simulink model "evap_simscape"  (R2023b)
settings: Solver=VariableStepAuto  StartTime=0.0  StopTime=eTime  RelTol=1e-3
values from neighbouring files (symbols this model uses):
  initial = struct()    [evap_simscape_code.m]
undefined symbols (not defined in the file or in its folder): refProp
libraries: nesl_utility x39, fl_lib x24, SimscapeFluids_lib x3
settings Model: Creator=jisung  LastModifiedBy=jisung
settings OptimizationCC: OptimizeBlockIOStorage=off  OptimizeDataStoreBuffers=off  BusAssignmentInplaceUpdate=off
settings DebuggingCC: SFUnexpectedBacktrackingDiag=warning  SFNoUnconditionalDefaultTransitionDiag=warning
settings RTWCC: GenCodeOnly=on  GenerateReport=on  Toolchain=Microsoft Visual C++ 2022 v17.0 | nmake (64-bit Windows)  BuildConfiguration=Debug  LaunchReport=on  TargetLang=C++
settings CodeAppCC: ForceParamTrailComments=on  MATLABSourceComments=on  EnableCustomComments=on
settings GRTTargetCC: TargetLangStandard=C++11 (ISO)  CombineSignalStateStructs=on  CodeInterfacePackaging=Reusable function  SupportVariableSizeSignals=on  GenerateAllocFcn=on  MultiInstanceErrorCode=Warning

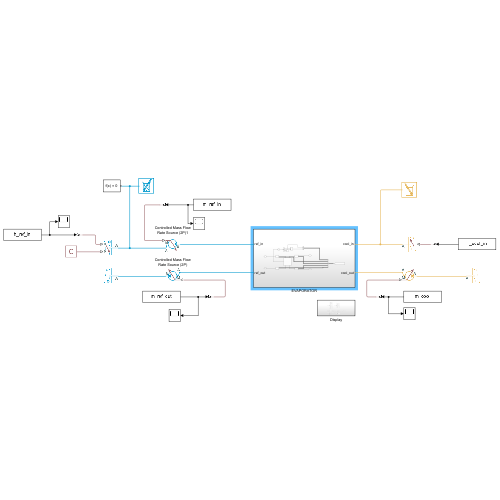
[thumbnail: Simulink's stored preview of the top-level diagram]
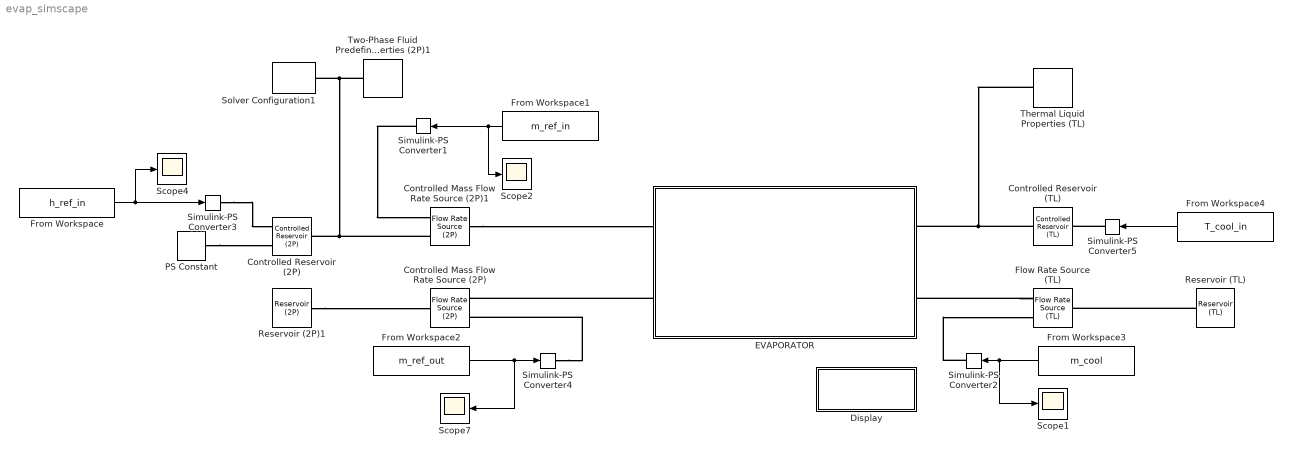
== system evap_simscape ==
  Controlled Mass Flow Rate Source (2P) : fl_lib/Two-Phase Fluid/Sources/Flow Rate Source (2P)  source_type=foundation.enum.constant_controlled.controlled  flow_type=foundation.enum.mass_volumetric_flow.mass  mass_flow=0 kg/s  volumetric_flow=0 m^3/s  power_spec=foundation.enum.power_spec.isentropic  area_A=pi * 12^2 / 4 mm^2  area_B=pi * 12^2 / 4 mm^2
      settings: InternalSimscapePortConfiguration="{\"Bottom\":[],\"Left\":[{\"id\":\"A\",\"label\":\"A\",\"type\":\"foundation.two_phase_fluid.two_phase_fluid\"},{\"id\":\"M\",\"label\":\"M\",\"type\":\"input\"}],\"Right\":[{\"id\":\"B\",\"label\":\"B\",\"type\":\"foundation.two_phase_fluid.two_phase_fluid\"}],\"Top\":[]}"
  Controlled Mass Flow Rate Source (2P)1 : fl_lib/Two-Phase Fluid/Sources/Flow Rate Source (2P)  source_type=foundation.enum.constant_controlled.controlled  flow_type=foundation.enum.mass_volumetric_flow.mass  mass_flow=0 kg/s  volumetric_flow=0 m^3/s  power_spec=foundation.enum.power_spec.isentropic  area_A=pi * 12^2 / 4 mm^2  area_B=pi * 12^2 / 4 mm^2
      settings: InternalSimscapePortConfiguration="{\"Bottom\":[],\"Left\":[{\"id\":\"A\",\"label\":\"A\",\"type\":\"foundation.two_phase_fluid.two_phase_fluid\"},{\"id\":\"M\",\"label\":\"M\",\"type\":\"input\"}],\"Right\":[{\"id\":\"B\",\"label\":\"B\",\"type\":\"foundation.two_phase_fluid.two_phase_fluid\"}],\"Top\":[]}"
  Controlled Reservoir (2P) : fl_lib/Two-Phase Fluid/Elements/Controlled Reservoir (2P)  pressure_spec=foundation.enum.ControlledReservoirPressureSpec2P.Specified  energy_spec=foundation.enum.ControlledReservoirEnergySpec2P.Enthalpy  area_A=0.01 m^2  pressure_limit_spec=foundation.enum.PressureLimitSpec2P.Warn
      settings: InternalSimscapePortConfiguration="{\"Bottom\":[],\"Left\":[{\"id\":\"A\",\"label\":\"A\",\"type\":\"foundation.two_phase_fluid.two_phase_fluid\"}],\"Right\":[{\"id\":\"H\",\"label\":\"H\",\"type\":\"input\"},{\"id\":\"P\",\"label\":\"P\",\"type\":\"input\"}],\"Top\":[]}"
  Controlled Reservoir (TL) : fl_lib/Thermal Liquid/Elements/Controlled Reservoir (TL)  pressure_spec=foundation.enum.pressure_spec.atmospheric  reservoir_pressure=0.101325 MPa  area=0.01 m^2
      settings: InternalSimscapePortConfiguration="{\"Bottom\":[],\"Left\":[{\"id\":\"A\",\"label\":\"A\",\"type\":\"foundation.thermal_liquid.thermal_liquid\"}],\"Right\":[{\"id\":\"T_in\",\"label\":\"T\",\"type\":\"input\"}],\"Top\":[]}"
  Display : Subsystem
  EVAPORATOR : Subsystem
  Flow Rate Source (TL) : fl_lib/Thermal Liquid/Sources/Flow Rate Source (TL)  source_type=foundation.enum.constant_controlled.controlled  flow_type=foundation.enum.mass_volumetric_flow.mass  mass_flow=0 kg/s  volumetric_flow=0 m^3/s  power_spec=foundation.enum.power_spec.isentropic  area=0.01 m^2
  From Workspace : FromWorkspace  VariableName=h_ref_in  Interpolate=off  OutputAfterFinalValue=Holding final value
  From Workspace1 : FromWorkspace  VariableName=m_ref_in  Interpolate=off  OutputAfterFinalValue=Holding final value
  From Workspace2 : FromWorkspace  VariableName=m_ref_out  Interpolate=off  OutputAfterFinalValue=Holding final value
  From Workspace3 : FromWorkspace  VariableName=m_cool  Interpolate=off  OutputAfterFinalValue=Holding final value
  From Workspace4 : FromWorkspace  VariableName=T_cool_in  Interpolate=off  OutputAfterFinalValue=Holding final value
  PS Constant : fl_lib/Physical Signals/Sources/PS Constant  constant=101.325 kPa
  Reservoir (2P)1 : fl_lib/Two-Phase Fluid/Elements/Reservoir (2P)  pressure_spec=foundation.enum.ReservoirPressureSpec2P.Specified  reservoir_pressure=400 kPa  reservoir_condensing_temperature=373.15 K  reservoir_evaporating_temperature=373.15 K  energy_spec=foundation.enum.ReservoirEnergySpec2P.Enthalpy  reservoir_temperature=ref_T_out degC  reservoir_quality=0  reservoir_void_fraction=0.5  reservoir_enthalpy=400 kJ/kg  reservoir_internal_energy=1500 kJ/kg  reservoir_subcooling=5 deltaK  reservoir_superheating=5 deltaK  area_A=0.01 m^2
  Reservoir (TL) : fl_lib/Thermal Liquid/Elements/Reservoir (TL)  pressure_spec=foundation.enum.pressure_spec.specified  reservoir_pressure=101.325 kPa  reservoir_temperature=initial.T_cool_in degC  area=0.01 m^2
  Scope{1..2,4,7} (4 alike) : Scope
  Simulink-PS Converter1 : nesl_utility/Simulink-PS Converter  PhysicalDomain=network_engine_domain  SubClassName=ps_input  LeftPortType=input  RightPortType=output  PseudoPeriodic=off  Frequencies=[]  NoiseDistribution=none  NoiseParameters=[]  Unit=kg/s  AffineConversion=off  FilteringAndDerivatives=provide  SimscapeFilterOrder=1  InputFilterTimeConstant=0.001  UdotUserProvided=0
  Simulink-PS Converter2 : nesl_utility/Simulink-PS Converter  PhysicalDomain=network_engine_domain  SubClassName=ps_input  LeftPortType=input  RightPortType=output  PseudoPeriodic=off  Frequencies=[]  NoiseDistribution=none  NoiseParameters=[]  Unit=kg/s  AffineConversion=off  FilteringAndDerivatives=provide  SimscapeFilterOrder=1  InputFilterTimeConstant=0.001  UdotUserProvided=0
  Simulink-PS Converter3 : nesl_utility/Simulink-PS Converter  PhysicalDomain=network_engine_domain  SubClassName=ps_input  LeftPortType=input  RightPortType=output  PseudoPeriodic=off  Frequencies=[]  NoiseDistribution=none  NoiseParameters=[]  Unit=kJ/kg  AffineConversion=off  FilteringAndDerivatives=provide  SimscapeFilterOrder=1  InputFilterTimeConstant=0.001  UdotUserProvided=0
  Simulink-PS Converter4 : nesl_utility/Simulink-PS Converter  PhysicalDomain=network_engine_domain  SubClassName=ps_input  LeftPortType=input  RightPortType=output  PseudoPeriodic=off  Frequencies=[]  NoiseDistribution=none  NoiseParameters=[]  Unit=kg/s  AffineConversion=off  FilteringAndDerivatives=provide  SimscapeFilterOrder=1  InputFilterTimeConstant=0.001  UdotUserProvided=0
  Simulink-PS Converter5 : nesl_utility/Simulink-PS Converter  PhysicalDomain=network_engine_domain  SubClassName=ps_input  LeftPortType=input  RightPortType=output  PseudoPeriodic=off  Frequencies=[]  NoiseDistribution=none  NoiseParameters=[]  Unit=degC  AffineConversion=on  FilteringAndDerivatives=provide  SimscapeFilterOrder=1  InputFilterTimeConstant=0.001  UdotUserProvided=0
  Solver Configuration1 : nesl_utility/Solver Configuration  PhysicalDomain=network_engine_domain  SubClassName=solver  LeftPortType=input  RightPortType=generic  Tones=[]  Harmonics=[]  SimulateNoise=off  Profile=off  UseLocalSampling=off  EnableSwitchedLinearOptims=on  FrequencyDomain=off  UseCCode=off  RelTol=0.001  AbsTol=1e-06  MinStep=1e-09  ToWorkspace=off  RevertToSquareIcSolve=off  NumHomotopyIterations=100  PhasorMode=off  PhasorModeNumHarmonics=1  ConsistencySolver=NEWTON_XTOL_AFTER_FTOL  IndexReductionMethod=DerivativeReplacement  DoDC=off  ResidualTolerance=1e-9  ConsistencyTolSource=GLOBAL  ConsistencyAbsTol=0.001  ConsistencyRelTol=0.001  ConsistencyTolFactor=0.001  UseLocalSolver=off  LocalSolverChoice=NE_BACKWARD_EULER_ADVANCER  ResolveIndetEquations=on  FunctionEvalNumThread=1  LocalSolverSampleTime=1  DoFixedCost=off  MaxNonlinIter=3  MaxModeIter=2  ComputeImpulses=off  ImpulseIterations=2  LinearAlgebra=auto  LinearAlgebraNumThread=0  EquationFormulation=NE_TIME_EF  DelaysMemoryBudget=1024  AutomaticFiltering=on  FilteringTimeConstant=0.001  PartitionStorageMethod=AS_NEEDED  PartitionMemoryBudget=1024  PartitionMethod=ROBUST  MultibodyUseLocalSolver=off  MultibodyLocalSolverChoice=ODE1  MultibodyLocalSolverSampleTime=0.001
  Thermal Liquid Properties (TL) : SimscapeFluids_lib/Thermal Liquid/Utilities/Thermal Liquid Properties (TL)  fluid_list=fluids.thermal_liquid.utilities.enum.thermal_liquid_fluid_list.ethylene_glycol  concentration_param_EG=fluids.thermal_liquid.utilities.enum.thermal_liquid_concentration.volume_fraction  concentration_param_PG=fluids.thermal_liquid.utilities.enum.thermal_liquid_concentration.volume_fraction  c_mass_SW=3.5e-3  c_mass_EG=0.1  c_mass_PG=0.1  c_mass_GL=0.1  c_vol_EG=0.5  c_vol_PG=0.1  beta_const_EG=2.1791 GPa  beta_const_PG=2.1791 GPa  beta_const_GL=2.1791 GPa  p_min_EG=0.01 MPa  p_min_PG=0.01 MPa  p_min_GL=0.01 MPa  p_max_EG=50 MPa  p_max_PG=50 MPa  p_max_GL=50 MPa  p_atm=0.101325 MPa  properties_range_check=simscape.enum.assert.action.error
  Two-Phase Fluid Predefined Properties (2P)1 : SimscapeFluids_lib/Two-Phase Fluid/Utilities/Two-Phase Fluid Predefined Properties (2P)  fluid=fluids.two_phase_fluid.utilities.enum.Fluid.R1234yf  p_atm=101.325 kPa  properties_range_check=simscape.enum.assert.action.error  q_rev=0.01 Pa
  wires:
  From Workspace/1 -> Scope4/1, Simulink-PS Converter3/1
  From Workspace2/1 -> Simulink-PS Converter4/1, Scope7/1
  From Workspace3/1 -> Scope1/1, Simulink-PS Converter2/1
  From Workspace4/1 -> Simulink-PS Converter5/1
  From Workspace1/1 -> Simulink-PS Converter1/1, Scope2/1
  connections:
  Reservoir (2P)1/LConn1 -- Controlled Mass Flow Rate Source (2P)/RConn1
  EVAPORATOR/RConn2 -- Controlled Mass Flow Rate Source (2P)/LConn1
  Simulink-PS Converter3/RConn1 -- Controlled Reservoir (2P)/RConn1
  Simulink-PS Converter4/RConn1 -- Controlled Mass Flow Rate Source (2P)/LConn2
  Reservoir (TL)/LConn1 -- Flow Rate Source (TL)/RConn1
  Controlled Reservoir (TL)/LConn1 -- Thermal Liquid Properties (TL)/RConn1 -- EVAPORATOR/LConn1
  Flow Rate Source (TL)/LConn1 -- EVAPORATOR/LConn2
  Simulink-PS Converter2/RConn1 -- Flow Rate Source (TL)/LConn2
  Simulink-PS Converter5/RConn1 -- Controlled Reservoir (TL)/RConn1
  PS Constant/RConn1 -- Controlled Reservoir (2P)/RConn2
  Controlled Mass Flow Rate Source (2P)1/RConn1 -- EVAPORATOR/RConn1
  Simulink-PS Converter1/RConn1 -- Controlled Mass Flow Rate Source (2P)1/LConn2
  Two-Phase Fluid Predefined Properties (2P)1/RConn1 -- Controlled Reservoir (2P)/LConn1 -- Controlled Mass Flow Rate Source (2P)1/LConn1 -- Solver Configuration1/RConn1

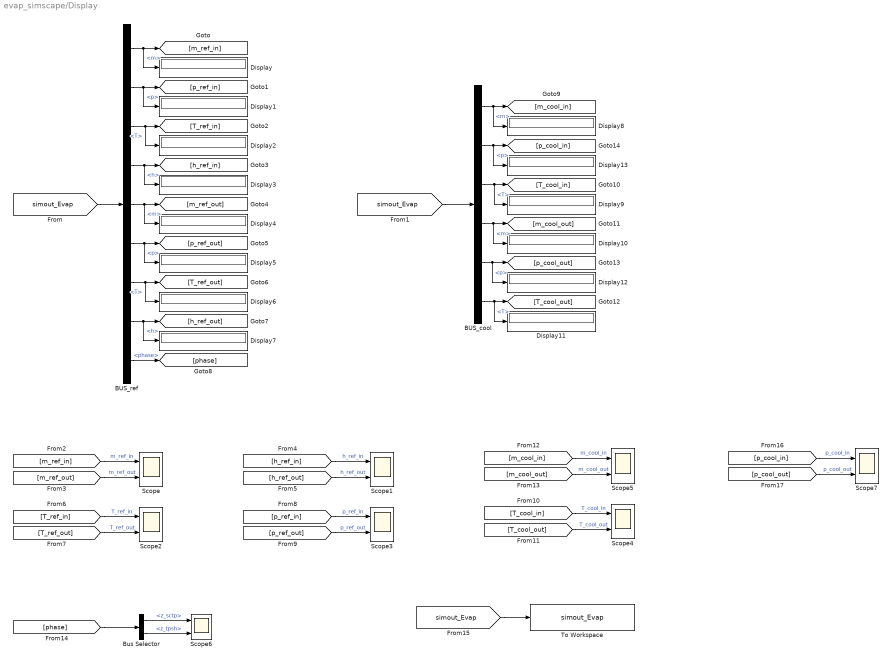
== system evap_simscape/Display ==
  BUS_cool : BusSelector  OutputSignals=cool_in.m,cool_in.p,cool_in.T,cool_out.m,cool_out.p,cool_out.T
  BUS_ref : BusSelector  OutputSignals=ref_in.m,ref_in.p,ref_in.T,ref_in.h,ref_out.m,ref_out.p,ref_out.T,ref_out.h,phase
  Bus Selector : BusSelector  OutputSignals=z_sctp,z_tpsh
  Display{,1..13} (14 alike) : Display
  Scope{,1..7} (8 alike) : Scope  NumInputPorts=2
  To Workspace : ToWorkspace  VariableName=simout_Evap  SaveFormat=Timeseries  SampleTime=-1
  wires:
  [simout_Evap] -> BUS_ref/1
  BUS_ref/1 -> Display/1, [m_ref_in]  "<m>"
  BUS_ref/2 -> Display1/1, [p_ref_in]  "<p>"
  BUS_ref/3 -> Display2/1, [T_ref_in]  "<T>"
  BUS_ref/4 -> Display3/1, [h_ref_in]  "<h>"
  BUS_ref/5 -> Display4/1, [m_ref_out]  "<m>"
  BUS_ref/6 -> Display5/1, [p_ref_out]  "<p>"
  BUS_ref/7 -> Display6/1, [T_ref_out]  "<T>"
  BUS_ref/8 -> Display7/1, [h_ref_out]  "<h>"
  BUS_ref/9 -> [phase]  "<phase>"
  [simout_Evap] -> BUS_cool/1
  BUS_cool/1 -> Display8/1, [m_cool_in]  "<m>"
  BUS_cool/3 -> Display9/1, [T_cool_in]  "<T>"
  BUS_cool/4 -> Display10/1, [m_cool_out]  "<m>"
  BUS_cool/6 -> Display11/1, [T_cool_out]  "<T>"
  [m_ref_in] -> Scope/1  "m_ref_in"
  [m_ref_out] -> Scope/2  "m_ref_out"
  [h_ref_out] -> Scope1/2  "h_ref_out"
  [h_ref_in] -> Scope1/1  "h_ref_in"
  [T_ref_out] -> Scope2/2  "T_ref_out"
  [T_ref_in] -> Scope2/1  "T_ref_in"
  [p_ref_out] -> Scope3/2  "p_ref_out"
  [p_ref_in] -> Scope3/1  "p_ref_in"
  [T_cool_out] -> Scope4/2  "T_cool_out"
  [T_cool_in] -> Scope4/1  "T_cool_in"
  [m_cool_out] -> Scope5/2  "m_cool_out"
  [m_cool_in] -> Scope5/1  "m_cool_in"
  [phase] -> Bus Selector/1
  [simout_Evap] -> To Workspace/1
  BUS_cool/5 -> Display12/1, [p_cool_out]  "<p>"
  BUS_cool/2 -> Display13/1, [p_cool_in]  "<p>"
  [p_cool_in] -> Scope7/1  "p_cool_in"
  [p_cool_out] -> Scope7/2  "p_cool_out"
  Bus Selector/1 -> Scope6/1  "<z_sctp>"
  Bus Selector/2 -> Scope6/2  "<z_tpsh>"

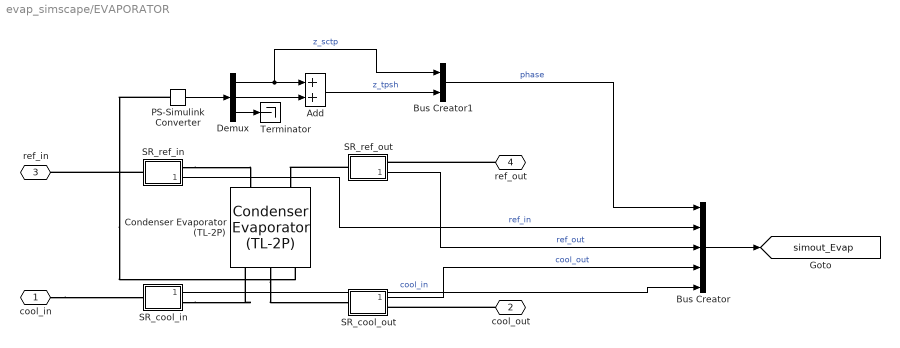
== system evap_simscape/EVAPORATOR ==
  Add : Sum
  Bus Creator : BusCreator  Inputs=5
  Bus Creator1 : BusCreator  Inputs=2
  Condenser Evaporator (TL-2P) : SimscapeFluids_lib/Fluid Network Interfaces/Heat Exchangers/Condenser Evaporator (TL-2P)  flow_arrangement=fluids.interfaces.heat_exchangers.enum.FlowArrangementTL2P.Counter  cross_flow_arrangement=fluids.interfaces.heat_exchangers.enum.CrossFlowArrangementTL2P.UnmixedUnmixed  R_wall=0 K/kW  area_A1=0.01 m^2  area_B1=0.01 m^2  area_A2=0.01 m^2  area_B2=0.01 m^2  flow_geometry_TL=fluids.interfaces.heat_exchangers.enum.FlowGeometryTL.InsideTubes  tube_num_TL=10  tube_length_TL=0.5 m  tube_cross_section_TL=fluids.interfaces.heat_exchangers.enum.TubeCrossSection.Rectangular  tube_diameter_TL=0.05 m  tube_width_TL=0.1 m  tube_height_TL=0.005 m  tube_inner_diameter_TL=0.05 m  tube_outer_diameter_TL=0.1 m  tube_flow_area_TL=0.002 m^2  tube_wetted_perimeter_TL=0.15 m  tube_heat_perimeter_TL=0.15 m  tube_pressure_loss_spec_TL=fluids.interfaces.heat_exchangers.enum.TubePressureLossSpec.LossCoeff  tube_loss_coeff_TL=125  tube_local_pressure_loss_spec_TL=fluids.thermal_liquid.pipes_fittings.enum.LocalLossSpec.AggregateLength  tube_length_add_TL=0.1 m  tube_local_loss_coefficient_TL=0.1  tube_roughness_pressure_TL=15e-6 m  tube_Re_lam_pressure_TL=2000  tube_Re_tur_pressure_TL=4000  tube_shape_factor_generic_TL=64  tube_heat_coeff_spec_TL=fluids.interfaces.heat_exchangers.enum.TubeHeatCoeffSpec.Colburn  tube_colburn_coeff_TL=[0.0861, .8, .33]  tube_roughness_heat_TL=15e-6 m  tube_Re_lam_heat_TL=2000  tube_Re_tur_heat_TL=4000  tube_Nu_lam_generic_TL=3.66  bank_arrangement_TL=fluids.interfaces.heat_exchangers.enum.BankArrangement.Inline  bank_num_rows_TL=6  bank_tubes_per_row_TL=6  bank_width_TL=1 m  bank_tube_diameter_TL=0.055 m  bank_longitudinal_pitch_TL=0.15 m  bank_transverse_pitch_TL=0.15 m  bank_pressure_loss_spec_TL=fluids.interfaces.heat_exchangers.enum.BankPressureLossSpec.Martin  bank_euler_TL=10  bank_heat_coeff_spec_TL=fluids.interfaces.heat_exchangers.enum.BankHeatCoeffSpec.Martin  bank_colburn_coeff_TL=[.27, .63, .36]  generic_flow_area_TL=0.01 m^2  generic_heat_area_TL=2 m^2  generic_volume_TL=0.05 m^3  generic_loss_coeff_TL=10  generic_colburn_coeff_TL=[.023, .8, .33]  fouling_factor_TL=0.1 K*m^2/kW  fin_area_TL=0 m^2  fin_efficiency_TL=0.5  p_init_TL=initial.p_cool kPa  T_init_TL=initial.T_cool_in degC  tube_num_2P=10  tube_length_2P=0.5 m  tube_cross_section_2P=fluids.interfaces.heat_exchangers.enum.TubeCrossSection.Rectangular  tube_diameter_2P=0.05 m  tube_width_2P=0.1 m  tube_height_2P=0.005 m  tube_inner_diameter_2P=0.05 m  tube_outer_diameter_2P=0.1 m  tube_flow_area_2P=0.002 m^2  tube_wetted_perimeter_2P=0.15 m  tube_heat_perimeter_2P=0.15 m  tube_pressure_loss_spec_2P=fluids.interfaces.heat_exchangers.enum.TubePressureLossSpec2P.LossCoeff  tube_loss_coeff_2P=125  tube_local_pressure_loss_spec_2P=fluids.two_phase_fluid.pipes_fittings.enum.LocalLossSpec.AggregateLength  tube_length_add_2P=0.1 m  tube_local_loss_coefficient_2P=0.1  tube_roughness_pressure_2P=15e-6 m  tube_Re_lam_pressure_2P=2000  tube_Re_tur_pressure_2P=4000  tube_shape_factor_generic_2P=64  tube_heat_coeff_spec_2P=fluids.interfaces.heat_exchangers.enum.TubeHeatCoeffSpec2P.Colburn  tube_colburn_coeff_liq_2P=[.023, .8, .33]  tube_colburn_coeff_mix_2P=[.280, .8, .33]  tube_colburn_coeff_vap_2P=[.023, .8, .33]  tube_roughness_heat_2P=15e-6 m  tube_Re_lam_heat_2P=2000  tube_Re_tur_heat_2P=4000  tube_Nu_lam_generic_2P=3.66  fouling_factor_2P=0.1 K*m^2/kW  fin_area_2P=0 m^2  fin_efficiency_2P=0.5  energy_spec_2P=foundation.enum.energy_spec.quality  p_init_2P=initial.pressure kPa  T_init_2P=-5 degC  x_init_2P=initial.quality  alpha_init_2P=0.5  h_init_2P=(refProp.vap_Hsat(initial.p_low) + refProp.liq_Hsat(initial.p_low)) / 2 kJ/kg  u_init_2P=1500 kJ/kg
      settings: InternalSimscapePortConfiguration="{\"Bottom\":[],\"Left\":[{\"id\":\"A1\",\"label\":\"A1\",\"type\":\"foundation.thermal_liquid.thermal_liquid\"},{\"id\":\"B1\",\"label\":\"B1\",\"type\":\"foundation.thermal_liquid.thermal_liquid\"}],\"Right\":[{\"id\":\"A2\",\"label\":\"A2\",\"type\":\"foundation.two_phase_fluid.two_phase_fluid\"},{\"id\":\"B2\",\"label\":\"B2\",\"type\":\"foundation.two_phase_fluid.two_phase_fluid\"}],\"Top\":[{\"id\":\"Z\",\"label\":\"Z\",\"type\":\"output\"}]}"
  Demux : Demux  Outputs=3
  PS-Simulink Converter : nesl_utility/PS-Simulink Converter  PhysicalDomain=network_engine_domain  SubClassName=ps_output  LeftPortType=input  RightPortType=output  PseudoPeriodic=off  Frequencies=[]  VectorFormat=1-D array  Unit=1  AffineConversion=off
  SR_cool_in : Subsystem
      mask Display: disp("SR")
  SR_cool_out : Subsystem
      mask Display: disp("SR")
  SR_ref_in : Subsystem
      settings: PortSchema="{\"entries\":[{\"content\":{\"sides\":[{\"content\":{\"connectorIds\":[\"LConn1\"]},\"type\":\"ConnectorPlacement.EquallySpacedRectSide\",\"uuid\":\"f46da1e2-6ace-4bb1-b592-c3f638213600\"},{\"content\":{\"connectorIds\":[\"RConn1\",\"Out1\"],\"side\":\"RIGHT\"},\"type\":\"ConnectorPlacement.EquallySpacedRectSide\",\"uuid\":\"b4f7967e-3f35-420b-953f-d92139738eaf\"},{\"content\":{\"side\":\"TOP\"},\"type\":\"ConnectorPlacement.EquallySpacedRectSide\",\"uuid\":\"c66c7f76-a790-428d-b4c7-3adf5f244887\"}]},\"type\":\"ConnectorPlacement.EquallySpacedConnector\",\"uuid\":\"beb29582-1898-4354-af88-a237db9df0a5\"}],\"packageUris\":[\"http://schema.mathworks.com/mf0/Connector/R2020b\"],\"version\":\"1.0\"}"
      mask Display: disp("SR")
  SR_ref_out : Subsystem
      settings: PortSchema="{\"entries\":[{\"content\":{\"sides\":[{\"content\":{\"connectorIds\":[\"LConn1\"]},\"type\":\"ConnectorPlacement.EquallySpacedRectSide\",\"uuid\":\"7b7e33ba-7b92-46b2-8bde-8aac1e6823e1\"},{\"content\":{\"connectorIds\":[\"RConn1\",\"Out1\"],\"side\":\"RIGHT\"},\"type\":\"ConnectorPlacement.EquallySpacedRectSide\",\"uuid\":\"bc058ced-a063-4dc0-960d-d036c5315ae1\"},{\"content\":{\"side\":\"TOP\"},\"type\":\"ConnectorPlacement.EquallySpacedRectSide\",\"uuid\":\"332fc07a-236e-4a4a-9036-d85954681cb2\"}]},\"type\":\"ConnectorPlacement.EquallySpacedConnector\",\"uuid\":\"69343ebb-29ec-4b9b-af1a-37b468795ca6\"}],\"packageUris\":[\"http://schema.mathworks.com/mf0/Connector/R2020b\"],\"version\":\"1.0\"}"
      mask Display: disp("SR")
  Terminator : Terminator
  cool_in : PMIOPort  Side=Left
  cool_out : PMIOPort  Port=2  Side=Left
  ref_in : PMIOPort  Port=3  Side=Right
  ref_out : PMIOPort  Port=4  Side=Right
  tag scope: simout_Evap=global
  wires:
  SR_cool_in/1(Coolant to evaporator out) -> Bus Creator/5  "cool_in"
  SR_ref_out/1(Refrigerant to compressor out) -> Bus Creator/3  "ref_out"
  SR_ref_in/1(Refrigerant to evaporator out) -> Bus Creator/2  "ref_in"
  SR_cool_out/1(Coolant from evaporator out) -> Bus Creator/4  "cool_out"
  Bus Creator/1 -> [simout_Evap]
  PS-Simulink Converter/1 -> Demux/1
  Demux/3 -> Terminator/1
  Demux/2 -> Add/2
  Add/1 -> Bus Creator1/2  "z_tpsh"
  Demux/1 -> Bus Creator1/1, Add/1  "z_sctp"
  Bus Creator1/1 -> Bus Creator/1  "phase"
  connections:
  ref_out/RConn1 -- SR_ref_out/RConn1
  SR_ref_in/LConn1 -- ref_in/RConn1
  cool_in/RConn1 -- SR_cool_in/LConn1
  SR_cool_in/RConn1 -- Condenser Evaporator (TL-2P)/LConn1
  Condenser Evaporator (TL-2P)/LConn2 -- SR_cool_out/LConn1
  SR_ref_out/LConn1 -- Condenser Evaporator (TL-2P)/RConn2
  SR_ref_in/RConn1 -- Condenser Evaporator (TL-2P)/RConn1
  PS-Simulink Converter/LConn1 -- Condenser Evaporator (TL-2P)/LConn3
  cool_out/RConn1 -- SR_cool_out/RConn1

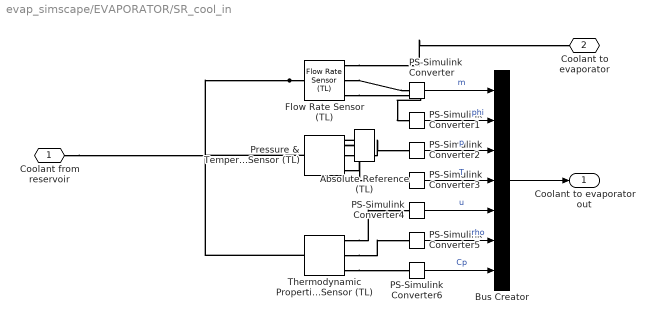
== system evap_simscape/EVAPORATOR/SR_cool_in ==
  Absolute Reference (TL) : fl_lib/Thermal Liquid/Elements/Absolute Reference (TL)
  Bus Creator : BusCreator  Inputs=7
  Flow Rate Sensor (TL) : fl_lib/Thermal Liquid/Sensors/Flow Rate Sensor (TL)  mass_flow_measure=true  volumetric_flow_measure=false  energy_flow_measure=true
      settings: InternalSimscapePortConfiguration="{\"Bottom\":[{\"id\":\"PHI\",\"label\":\"φ\",\"type\":\"output\"}],\"Left\":[{\"id\":\"A\",\"label\":\"A\",\"type\":\"foundation.thermal_liquid.thermal_liquid\"}],\"Right\":[{\"id\":\"B\",\"label\":\"B\",\"type\":\"foundation.thermal_liquid.thermal_liquid\"},{\"id\":\"M\",\"label\":\"M\",\"type\":\"output\"}],\"Top\":[]}"
  PS-Simulink Converter : nesl_utility/PS-Simulink Converter  PhysicalDomain=network_engine_domain  SubClassName=ps_output  LeftPortType=input  RightPortType=output  PseudoPeriodic=off  Frequencies=[]  VectorFormat=1-D array  Unit=kg/s  AffineConversion=off
  PS-Simulink Converter1 : nesl_utility/PS-Simulink Converter  PhysicalDomain=network_engine_domain  SubClassName=ps_output  LeftPortType=input  RightPortType=output  PseudoPeriodic=off  Frequencies=[]  VectorFormat=1-D array  Unit=kW  AffineConversion=off
  PS-Simulink Converter2 : nesl_utility/PS-Simulink Converter  PhysicalDomain=network_engine_domain  SubClassName=ps_output  LeftPortType=input  RightPortType=output  PseudoPeriodic=off  Frequencies=[]  VectorFormat=1-D array  Unit=kPa  AffineConversion=off
  PS-Simulink Converter3 : nesl_utility/PS-Simulink Converter  PhysicalDomain=network_engine_domain  SubClassName=ps_output  LeftPortType=input  RightPortType=output  PseudoPeriodic=off  Frequencies=[]  VectorFormat=1-D array  Unit=degC  AffineConversion=on
  PS-Simulink Converter4 : nesl_utility/PS-Simulink Converter  PhysicalDomain=network_engine_domain  SubClassName=ps_output  LeftPortType=input  RightPortType=output  PseudoPeriodic=off  Frequencies=[]  VectorFormat=1-D array  Unit=kJ/kg  AffineConversion=off
  PS-Simulink Converter5 : nesl_utility/PS-Simulink Converter  PhysicalDomain=network_engine_domain  SubClassName=ps_output  LeftPortType=input  RightPortType=output  PseudoPeriodic=off  Frequencies=[]  VectorFormat=1-D array  Unit=kg/m^3  AffineConversion=off
  PS-Simulink Converter6 : nesl_utility/PS-Simulink Converter  PhysicalDomain=network_engine_domain  SubClassName=ps_output  LeftPortType=input  RightPortType=output  PseudoPeriodic=off  Frequencies=[]  VectorFormat=1-D array  Unit=kJ/(kg*K)  AffineConversion=off
  Pressure & Temperature Sensor (TL) : fl_lib/Thermal Liquid/Sensors/Pressure & Temperature Sensor (TL)  reference=foundation.enum.MeasurementReference.difference  pressure=true  pressure_spec=foundation.enum.PressureMeasementSpec.Absolute  temperature=true
      settings: InternalSimscapePortConfiguration="{\"Bottom\":[{\"id\":\"T\",\"label\":\"T\",\"type\":\"output\"}],\"Left\":[{\"id\":\"A\",\"label\":\"A\",\"type\":\"foundation.thermal_liquid.thermal_liquid\"}],\"Right\":[{\"id\":\"B\",\"label\":\"B\",\"type\":\"foundation.thermal_liquid.thermal_liquid\"},{\"id\":\"P\",\"label\":\"P\",\"type\":\"output\"}],\"Top\":[]}"
  Thermodynamic Properties Sensor (TL) : fl_lib/Thermal Liquid/Sensors/Thermodynamic Properties Sensor (TL)  internal_energy=true  density=true  specific_heat=true
      settings: InternalSimscapePortConfiguration="{\"Bottom\":[],\"Left\":[{\"id\":\"A\",\"label\":\"A\",\"type\":\"foundation.thermal_liquid.thermal_liquid\"}],\"Right\":[{\"id\":\"U\",\"label\":\"u\",\"type\":\"output\"},{\"id\":\"RHO\",\"label\":\"ρ\",\"type\":\"output\"},{\"id\":\"CP\",\"label\":\"cp\",\"type\":\"output\"}],\"Top\":[]}"
  " Coolant from reservoir" : PMIOPort  Side=Left
  " Coolant to evaporator" : PMIOPort  Port=2  Side=Right
  Coolant to evaporator out : Outport
  wires:
  PS-Simulink Converter/1 -> Bus Creator/1  "m"
  PS-Simulink Converter1/1 -> Bus Creator/2  "phi"
  PS-Simulink Converter2/1 -> Bus Creator/3  "p"
  PS-Simulink Converter3/1 -> Bus Creator/4  "T"
  PS-Simulink Converter4/1 -> Bus Creator/5  "u"
  PS-Simulink Converter5/1 -> Bus Creator/6  "rho"
  PS-Simulink Converter6/1 -> Bus Creator/7  "Cp"
  Bus Creator/1 -> Coolant to evaporator out/1
  connections:
  Flow Rate Sensor (TL)/LConn1 -- " Coolant from reservoir"/RConn1 -- Pressure & Temperature Sensor (TL)/LConn1 -- Thermodynamic Properties Sensor (TL)/LConn1
  Flow Rate Sensor (TL)/RConn1 -- " Coolant to evaporator"/RConn1
  Absolute Reference (TL)/LConn1 -- Pressure & Temperature Sensor (TL)/RConn1
  Flow Rate Sensor (TL)/RConn2 -- PS-Simulink Converter/LConn1
  Flow Rate Sensor (TL)/RConn3 -- PS-Simulink Converter1/LConn1
  Pressure & Temperature Sensor (TL)/RConn2 -- PS-Simulink Converter2/LConn1
  Pressure & Temperature Sensor (TL)/RConn3 -- PS-Simulink Converter3/LConn1
  Thermodynamic Properties Sensor (TL)/RConn1 -- PS-Simulink Converter4/LConn1
  Thermodynamic Properties Sensor (TL)/RConn2 -- PS-Simulink Converter5/LConn1
  Thermodynamic Properties Sensor (TL)/RConn3 -- PS-Simulink Converter6/LConn1

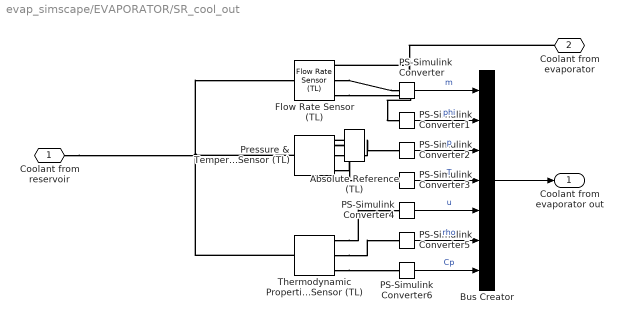
== system evap_simscape/EVAPORATOR/SR_cool_out ==
  Absolute Reference (TL) : fl_lib/Thermal Liquid/Elements/Absolute Reference (TL)
  Bus Creator : BusCreator  Inputs=7
  Flow Rate Sensor (TL) : fl_lib/Thermal Liquid/Sensors/Flow Rate Sensor (TL)  mass_flow_measure=true  volumetric_flow_measure=false  energy_flow_measure=true
      settings: InternalSimscapePortConfiguration="{\"Bottom\":[{\"id\":\"PHI\",\"label\":\"φ\",\"type\":\"output\"}],\"Left\":[{\"id\":\"A\",\"label\":\"A\",\"type\":\"foundation.thermal_liquid.thermal_liquid\"}],\"Right\":[{\"id\":\"B\",\"label\":\"B\",\"type\":\"foundation.thermal_liquid.thermal_liquid\"},{\"id\":\"M\",\"label\":\"M\",\"type\":\"output\"}],\"Top\":[]}"
  PS-Simulink Converter : nesl_utility/PS-Simulink Converter  PhysicalDomain=network_engine_domain  SubClassName=ps_output  LeftPortType=input  RightPortType=output  PseudoPeriodic=off  Frequencies=[]  VectorFormat=1-D array  Unit=kg/s  AffineConversion=off
  PS-Simulink Converter1 : nesl_utility/PS-Simulink Converter  PhysicalDomain=network_engine_domain  SubClassName=ps_output  LeftPortType=input  RightPortType=output  PseudoPeriodic=off  Frequencies=[]  VectorFormat=1-D array  Unit=kW  AffineConversion=off
  PS-Simulink Converter2 : nesl_utility/PS-Simulink Converter  PhysicalDomain=network_engine_domain  SubClassName=ps_output  LeftPortType=input  RightPortType=output  PseudoPeriodic=off  Frequencies=[]  VectorFormat=1-D array  Unit=kPa  AffineConversion=off
  PS-Simulink Converter3 : nesl_utility/PS-Simulink Converter  PhysicalDomain=network_engine_domain  SubClassName=ps_output  LeftPortType=input  RightPortType=output  PseudoPeriodic=off  Frequencies=[]  VectorFormat=1-D array  Unit=degC  AffineConversion=on
  PS-Simulink Converter4 : nesl_utility/PS-Simulink Converter  PhysicalDomain=network_engine_domain  SubClassName=ps_output  LeftPortType=input  RightPortType=output  PseudoPeriodic=off  Frequencies=[]  VectorFormat=1-D array  Unit=kJ/kg  AffineConversion=off
  PS-Simulink Converter5 : nesl_utility/PS-Simulink Converter  PhysicalDomain=network_engine_domain  SubClassName=ps_output  LeftPortType=input  RightPortType=output  PseudoPeriodic=off  Frequencies=[]  VectorFormat=1-D array  Unit=kg/m^3  AffineConversion=off
  PS-Simulink Converter6 : nesl_utility/PS-Simulink Converter  PhysicalDomain=network_engine_domain  SubClassName=ps_output  LeftPortType=input  RightPortType=output  PseudoPeriodic=off  Frequencies=[]  VectorFormat=1-D array  Unit=kJ/(kg*K)  AffineConversion=off
  Pressure & Temperature Sensor (TL) : fl_lib/Thermal Liquid/Sensors/Pressure & Temperature Sensor (TL)  reference=foundation.enum.MeasurementReference.difference  pressure=true  pressure_spec=foundation.enum.PressureMeasementSpec.Absolute  temperature=true
      settings: InternalSimscapePortConfiguration="{\"Bottom\":[{\"id\":\"T\",\"label\":\"T\",\"type\":\"output\"}],\"Left\":[{\"id\":\"A\",\"label\":\"A\",\"type\":\"foundation.thermal_liquid.thermal_liquid\"}],\"Right\":[{\"id\":\"B\",\"label\":\"B\",\"type\":\"foundation.thermal_liquid.thermal_liquid\"},{\"id\":\"P\",\"label\":\"P\",\"type\":\"output\"}],\"Top\":[]}"
  Thermodynamic Properties Sensor (TL) : fl_lib/Thermal Liquid/Sensors/Thermodynamic Properties Sensor (TL)  internal_energy=true  density=true  specific_heat=true
      settings: InternalSimscapePortConfiguration="{\"Bottom\":[],\"Left\":[{\"id\":\"A\",\"label\":\"A\",\"type\":\"foundation.thermal_liquid.thermal_liquid\"}],\"Right\":[{\"id\":\"U\",\"label\":\"u\",\"type\":\"output\"},{\"id\":\"RHO\",\"label\":\"ρ\",\"type\":\"output\"},{\"id\":\"CP\",\"label\":\"cp\",\"type\":\"output\"}],\"Top\":[]}"
  " Coolant from reservoir" : PMIOPort  Side=Left
  " Coolant from evaporator" : PMIOPort  Port=2  Side=Right
  Coolant from evaporator out : Outport
  wires:
  Bus Creator/1 -> Coolant from evaporator out/1
  PS-Simulink Converter/1 -> Bus Creator/1  "m"
  PS-Simulink Converter4/1 -> Bus Creator/5  "u"
  PS-Simulink Converter2/1 -> Bus Creator/3  "p"
  PS-Simulink Converter5/1 -> Bus Creator/6  "rho"
  PS-Simulink Converter3/1 -> Bus Creator/4  "T"
  PS-Simulink Converter1/1 -> Bus Creator/2  "phi"
  PS-Simulink Converter6/1 -> Bus Creator/7  "Cp"
  connections:
  Thermodynamic Properties Sensor (TL)/LConn1 -- " Coolant from reservoir"/RConn1 -- Flow Rate Sensor (TL)/LConn1 -- Pressure & Temperature Sensor (TL)/LConn1
  Absolute Reference (TL)/LConn1 -- Pressure & Temperature Sensor (TL)/RConn1
  Thermodynamic Properties Sensor (TL)/RConn1 -- PS-Simulink Converter4/LConn1
  Pressure & Temperature Sensor (TL)/RConn2 -- PS-Simulink Converter2/LConn1
  " Coolant from evaporator"/RConn1 -- Flow Rate Sensor (TL)/RConn1
  Thermodynamic Properties Sensor (TL)/RConn3 -- PS-Simulink Converter6/LConn1
  Thermodynamic Properties Sensor (TL)/RConn2 -- PS-Simulink Converter5/LConn1
  Flow Rate Sensor (TL)/RConn3 -- PS-Simulink Converter1/LConn1
  Pressure & Temperature Sensor (TL)/RConn3 -- PS-Simulink Converter3/LConn1
  Flow Rate Sensor (TL)/RConn2 -- PS-Simulink Converter/LConn1

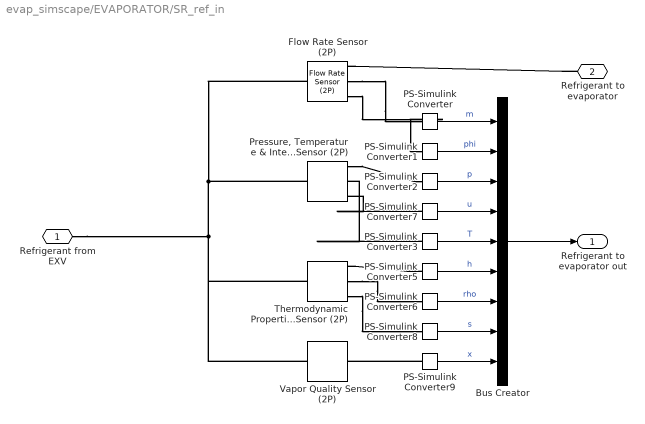
== system evap_simscape/EVAPORATOR/SR_ref_in ==
  Bus Creator : BusCreator  Inputs=9
  Flow Rate Sensor (2P) : fl_lib/Two-Phase Fluid/Sensors/Flow Rate Sensor (2P)  mass_flow_measure=true  volumetric_flow_measure=false  energy_flow_measure=true
      settings: InternalSimscapePortConfiguration="{\"Bottom\":[{\"id\":\"PHI\",\"label\":\"φ\",\"type\":\"output\"}],\"Left\":[{\"id\":\"A\",\"label\":\"A\",\"type\":\"foundation.two_phase_fluid.two_phase_fluid\"}],\"Right\":[{\"id\":\"B\",\"label\":\"B\",\"type\":\"foundation.two_phase_fluid.two_phase_fluid\"},{\"id\":\"M\",\"label\":\"M\",\"type\":\"output\"}],\"Top\":[]}"
  PS-Simulink Converter : nesl_utility/PS-Simulink Converter  PhysicalDomain=network_engine_domain  SubClassName=ps_output  LeftPortType=input  RightPortType=output  PseudoPeriodic=off  Frequencies=[]  VectorFormat=1-D array  Unit=kg/s  AffineConversion=off
  PS-Simulink Converter1 : nesl_utility/PS-Simulink Converter  PhysicalDomain=network_engine_domain  SubClassName=ps_output  LeftPortType=input  RightPortType=output  PseudoPeriodic=off  Frequencies=[]  VectorFormat=1-D array  Unit=kW  AffineConversion=off
  PS-Simulink Converter2 : nesl_utility/PS-Simulink Converter  PhysicalDomain=network_engine_domain  SubClassName=ps_output  LeftPortType=input  RightPortType=output  PseudoPeriodic=off  Frequencies=[]  VectorFormat=1-D array  Unit=kPa  AffineConversion=off
  PS-Simulink Converter3 : nesl_utility/PS-Simulink Converter  PhysicalDomain=network_engine_domain  SubClassName=ps_output  LeftPortType=input  RightPortType=output  PseudoPeriodic=off  Frequencies=[]  VectorFormat=1-D array  Unit=degC  AffineConversion=on
  PS-Simulink Converter5 : nesl_utility/PS-Simulink Converter  PhysicalDomain=network_engine_domain  SubClassName=ps_output  LeftPortType=input  RightPortType=output  PseudoPeriodic=off  Frequencies=[]  VectorFormat=1-D array  Unit=kJ/kg  AffineConversion=off
  PS-Simulink Converter6 : nesl_utility/PS-Simulink Converter  PhysicalDomain=network_engine_domain  SubClassName=ps_output  LeftPortType=input  RightPortType=output  PseudoPeriodic=off  Frequencies=[]  VectorFormat=1-D array  Unit=kg/m^3  AffineConversion=off
  PS-Simulink Converter7 : nesl_utility/PS-Simulink Converter  PhysicalDomain=network_engine_domain  SubClassName=ps_output  LeftPortType=input  RightPortType=output  PseudoPeriodic=off  Frequencies=[]  VectorFormat=1-D array  Unit=kJ/kg  AffineConversion=on
  PS-Simulink Converter8 : nesl_utility/PS-Simulink Converter  PhysicalDomain=network_engine_domain  SubClassName=ps_output  LeftPortType=input  RightPortType=output  PseudoPeriodic=off  Frequencies=[]  VectorFormat=1-D array  Unit=kJ/(kg*K)  AffineConversion=off
  PS-Simulink Converter9 : nesl_utility/PS-Simulink Converter  PhysicalDomain=network_engine_domain  SubClassName=ps_output  LeftPortType=input  RightPortType=output  PseudoPeriodic=off  Frequencies=[]  VectorFormat=1-D array  Unit=1  AffineConversion=off
  "Pressure, Temperature & Internal Energy Sensor (2P)" : fl_lib/Two-Phase Fluid/Sensors/Pressure, Temperature & Internal Energy Sensor (2P)  reference=foundation.enum.MeasurementReference.absolute  pressure=true  pressure_spec=foundation.enum.PressureMeasementSpec.Absolute  temperature=true  internal_energy=true
      settings: InternalSimscapePortConfiguration="{\"Bottom\":[{\"id\":\"T\",\"label\":\"T\",\"type\":\"output\"},{\"id\":\"U\",\"label\":\"U\",\"type\":\"output\"}],\"Left\":[{\"id\":\"A\",\"label\":\"A\",\"type\":\"foundation.two_phase_fluid.two_phase_fluid\"}],\"Right\":[{\"id\":\"Pa\",\"label\":\"Pa\",\"type\":\"output\"}],\"Top\":[]}"
  Thermodynamic Properties Sensor (2P) : fl_lib/Two-Phase Fluid/Sensors/Thermodynamic Properties Sensor (2P)  temperature=false  enthalpy=true  density=true  specific_volume=false  entropy=true
      settings: InternalSimscapePortConfiguration="{\"Bottom\":[{\"id\":\"S\",\"label\":\"s\",\"type\":\"output\"}],\"Left\":[{\"id\":\"A\",\"label\":\"A\",\"type\":\"foundation.two_phase_fluid.two_phase_fluid\"}],\"Right\":[{\"id\":\"H\",\"label\":\"h\",\"type\":\"output\"},{\"id\":\"RHO\",\"label\":\"ρ\",\"type\":\"output\"}],\"Top\":[]}"
  Vapor Quality Sensor (2P) : fl_lib/Two-Phase Fluid/Sensors/Vapor Quality Sensor (2P)  vapor_fraction_spec=foundation.enum.vapor_fraction_spec.quality
      settings: InternalSimscapePortConfiguration="{\"Bottom\":[],\"Left\":[{\"id\":\"A\",\"label\":\"A\",\"type\":\"foundation.two_phase_fluid.two_phase_fluid\"}],\"Right\":[{\"id\":\"X\",\"label\":\"X\",\"type\":\"output\"}],\"Top\":[]}"
  Refrigerant from EXV : PMIOPort  Side=Left
  " Refrigerant to evaporator" : PMIOPort  Port=2  Side=Right
  Refrigerant to evaporator out : Outport
  wires:
  Bus Creator/1 -> Refrigerant to evaporator out/1
  PS-Simulink Converter9/1 -> Bus Creator/9  "x"
  PS-Simulink Converter8/1 -> Bus Creator/8  "s"
  PS-Simulink Converter3/1 -> Bus Creator/5  "T"
  PS-Simulink Converter/1 -> Bus Creator/1  "m"
  PS-Simulink Converter7/1 -> Bus Creator/4  "u"
  PS-Simulink Converter1/1 -> Bus Creator/2  "phi"
  PS-Simulink Converter2/1 -> Bus Creator/3  "p"
  PS-Simulink Converter6/1 -> Bus Creator/7  "rho"
  PS-Simulink Converter5/1 -> Bus Creator/6  "h"
  connections:
  Flow Rate Sensor (2P)/LConn1 -- Refrigerant from EXV/RConn1 -- Vapor Quality Sensor (2P)/LConn1 -- Thermodynamic Properties Sensor (2P)/LConn1 -- "Pressure, Temperature & Internal Energy Sensor (2P)"/LConn1
  Flow Rate Sensor (2P)/RConn3 -- PS-Simulink Converter1/LConn1
  Thermodynamic Properties Sensor (2P)/RConn2 -- PS-Simulink Converter6/LConn1
  " Refrigerant to evaporator"/RConn1 -- Flow Rate Sensor (2P)/RConn1
  Thermodynamic Properties Sensor (2P)/RConn3 -- PS-Simulink Converter8/LConn1
  PS-Simulink Converter3/LConn1 -- "Pressure, Temperature & Internal Energy Sensor (2P)"/RConn2
  PS-Simulink Converter9/LConn1 -- Vapor Quality Sensor (2P)/RConn1
  "Pressure, Temperature & Internal Energy Sensor (2P)"/RConn1 -- PS-Simulink Converter2/LConn1
  PS-Simulink Converter7/LConn1 -- "Pressure, Temperature & Internal Energy Sensor (2P)"/RConn3
  Flow Rate Sensor (2P)/RConn2 -- PS-Simulink Converter/LConn1
  PS-Simulink Converter5/LConn1 -- Thermodynamic Properties Sensor (2P)/RConn1

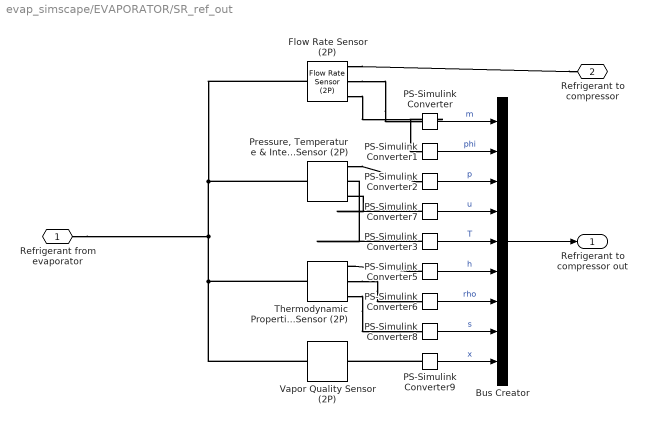
== system evap_simscape/EVAPORATOR/SR_ref_out ==
  Bus Creator : BusCreator  Inputs=9
  Flow Rate Sensor (2P) : fl_lib/Two-Phase Fluid/Sensors/Flow Rate Sensor (2P)  mass_flow_measure=true  volumetric_flow_measure=false  energy_flow_measure=true
      settings: InternalSimscapePortConfiguration="{\"Bottom\":[{\"id\":\"PHI\",\"label\":\"φ\",\"type\":\"output\"}],\"Left\":[{\"id\":\"A\",\"label\":\"A\",\"type\":\"foundation.two_phase_fluid.two_phase_fluid\"}],\"Right\":[{\"id\":\"B\",\"label\":\"B\",\"type\":\"foundation.two_phase_fluid.two_phase_fluid\"},{\"id\":\"M\",\"label\":\"M\",\"type\":\"output\"}],\"Top\":[]}"
  PS-Simulink Converter : nesl_utility/PS-Simulink Converter  PhysicalDomain=network_engine_domain  SubClassName=ps_output  LeftPortType=input  RightPortType=output  PseudoPeriodic=off  Frequencies=[]  VectorFormat=1-D array  Unit=kg/s  AffineConversion=off
  PS-Simulink Converter1 : nesl_utility/PS-Simulink Converter  PhysicalDomain=network_engine_domain  SubClassName=ps_output  LeftPortType=input  RightPortType=output  PseudoPeriodic=off  Frequencies=[]  VectorFormat=1-D array  Unit=kW  AffineConversion=off
  PS-Simulink Converter2 : nesl_utility/PS-Simulink Converter  PhysicalDomain=network_engine_domain  SubClassName=ps_output  LeftPortType=input  RightPortType=output  PseudoPeriodic=off  Frequencies=[]  VectorFormat=1-D array  Unit=kPa  AffineConversion=off
  PS-Simulink Converter3 : nesl_utility/PS-Simulink Converter  PhysicalDomain=network_engine_domain  SubClassName=ps_output  LeftPortType=input  RightPortType=output  PseudoPeriodic=off  Frequencies=[]  VectorFormat=1-D array  Unit=degC  AffineConversion=on
  PS-Simulink Converter5 : nesl_utility/PS-Simulink Converter  PhysicalDomain=network_engine_domain  SubClassName=ps_output  LeftPortType=input  RightPortType=output  PseudoPeriodic=off  Frequencies=[]  VectorFormat=1-D array  Unit=kJ/kg  AffineConversion=off
  PS-Simulink Converter6 : nesl_utility/PS-Simulink Converter  PhysicalDomain=network_engine_domain  SubClassName=ps_output  LeftPortType=input  RightPortType=output  PseudoPeriodic=off  Frequencies=[]  VectorFormat=1-D array  Unit=kg/m^3  AffineConversion=off
  PS-Simulink Converter7 : nesl_utility/PS-Simulink Converter  PhysicalDomain=network_engine_domain  SubClassName=ps_output  LeftPortType=input  RightPortType=output  PseudoPeriodic=off  Frequencies=[]  VectorFormat=1-D array  Unit=kJ/kg  AffineConversion=on
  PS-Simulink Converter8 : nesl_utility/PS-Simulink Converter  PhysicalDomain=network_engine_domain  SubClassName=ps_output  LeftPortType=input  RightPortType=output  PseudoPeriodic=off  Frequencies=[]  VectorFormat=1-D array  Unit=kJ/(kg*K)  AffineConversion=off
  PS-Simulink Converter9 : nesl_utility/PS-Simulink Converter  PhysicalDomain=network_engine_domain  SubClassName=ps_output  LeftPortType=input  RightPortType=output  PseudoPeriodic=off  Frequencies=[]  VectorFormat=1-D array  Unit=1  AffineConversion=off
  "Pressure, Temperature & Internal Energy Sensor (2P)" : fl_lib/Two-Phase Fluid/Sensors/Pressure, Temperature & Internal Energy Sensor (2P)  reference=foundation.enum.MeasurementReference.absolute  pressure=true  pressure_spec=foundation.enum.PressureMeasementSpec.Absolute  temperature=true  internal_energy=true
      settings: InternalSimscapePortConfiguration="{\"Bottom\":[{\"id\":\"T\",\"label\":\"T\",\"type\":\"output\"},{\"id\":\"U\",\"label\":\"U\",\"type\":\"output\"}],\"Left\":[{\"id\":\"A\",\"label\":\"A\",\"type\":\"foundation.two_phase_fluid.two_phase_fluid\"}],\"Right\":[{\"id\":\"Pa\",\"label\":\"Pa\",\"type\":\"output\"}],\"Top\":[]}"
  Thermodynamic Properties Sensor (2P) : fl_lib/Two-Phase Fluid/Sensors/Thermodynamic Properties Sensor (2P)  temperature=false  enthalpy=true  density=true  specific_volume=false  entropy=true
      settings: InternalSimscapePortConfiguration="{\"Bottom\":[{\"id\":\"S\",\"label\":\"s\",\"type\":\"output\"}],\"Left\":[{\"id\":\"A\",\"label\":\"A\",\"type\":\"foundation.two_phase_fluid.two_phase_fluid\"}],\"Right\":[{\"id\":\"H\",\"label\":\"h\",\"type\":\"output\"},{\"id\":\"RHO\",\"label\":\"ρ\",\"type\":\"output\"}],\"Top\":[]}"
  Vapor Quality Sensor (2P) : fl_lib/Two-Phase Fluid/Sensors/Vapor Quality Sensor (2P)  vapor_fraction_spec=foundation.enum.vapor_fraction_spec.quality
      settings: InternalSimscapePortConfiguration="{\"Bottom\":[],\"Left\":[{\"id\":\"A\",\"label\":\"A\",\"type\":\"foundation.two_phase_fluid.two_phase_fluid\"}],\"Right\":[{\"id\":\"X\",\"label\":\"X\",\"type\":\"output\"}],\"Top\":[]}"
  Refrigerant from evaporator : PMIOPort  Side=Left
  " Refrigerant to compressor" : PMIOPort  Port=2  Side=Right
  Refrigerant to compressor out : Outport
  wires:
  Bus Creator/1 -> Refrigerant to compressor out/1
  PS-Simulink Converter9/1 -> Bus Creator/9  "x"
  PS-Simulink Converter8/1 -> Bus Creator/8  "s"
  PS-Simulink Converter3/1 -> Bus Creator/5  "T"
  PS-Simulink Converter/1 -> Bus Creator/1  "m"
  PS-Simulink Converter7/1 -> Bus Creator/4  "u"
  PS-Simulink Converter1/1 -> Bus Creator/2  "phi"
  PS-Simulink Converter2/1 -> Bus Creator/3  "p"
  PS-Simulink Converter6/1 -> Bus Creator/7  "rho"
  PS-Simulink Converter5/1 -> Bus Creator/6  "h"
  connections:
  Flow Rate Sensor (2P)/LConn1 -- Refrigerant from evaporator/RConn1 -- Vapor Quality Sensor (2P)/LConn1 -- Thermodynamic Properties Sensor (2P)/LConn1 -- "Pressure, Temperature & Internal Energy Sensor (2P)"/LConn1
  Flow Rate Sensor (2P)/RConn3 -- PS-Simulink Converter1/LConn1
  Thermodynamic Properties Sensor (2P)/RConn2 -- PS-Simulink Converter6/LConn1
  Flow Rate Sensor (2P)/RConn1 -- " Refrigerant to compressor"/RConn1
  Thermodynamic Properties Sensor (2P)/RConn3 -- PS-Simulink Converter8/LConn1
  PS-Simulink Converter3/LConn1 -- "Pressure, Temperature & Internal Energy Sensor (2P)"/RConn2
  PS-Simulink Converter9/LConn1 -- Vapor Quality Sensor (2P)/RConn1
  "Pressure, Temperature & Internal Energy Sensor (2P)"/RConn1 -- PS-Simulink Converter2/LConn1
  PS-Simulink Converter7/LConn1 -- "Pressure, Temperature & Internal Energy Sensor (2P)"/RConn3
  Flow Rate Sensor (2P)/RConn2 -- PS-Simulink Converter/LConn1
  PS-Simulink Converter5/LConn1 -- Thermodynamic Properties Sensor (2P)/RConn1
